simulink model "untitled1_2"  (R2020a)
settings: Solver=VariableStepAuto  StartTime=0.0  StopTime=10.0  RelTol=1e-3
values from neighbouring files (symbols this model uses):
  th1 = 3.1    [Lab1.m]
  th2 = 9.5    [Lab1.m]
  th3 = 0.24    [Lab1.m]
  th4 = 0.77    [Lab1.m]
settings Model: Creator=ajankowi  LastModifiedBy=adamj

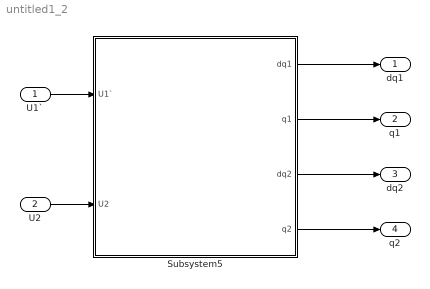
== system untitled1_2 ==
  U1` : Inport
  U2 : Inport  Port=2
  Subsystem5 : Subsystem
  dq1 : Outport
  q1 : Outport  Port=2
  dq2 : Outport  Port=3
  q2 : Outport  Port=4
  wires:
  U1`/1 -> Subsystem5/1(U1`)
  U2/1 -> Subsystem5/2(U2)
  Subsystem5/1(dq1) -> dq1/1
  Subsystem5/2(q1) -> q1/1
  Subsystem5/3(dq2) -> dq2/1
  Subsystem5/4(q2) -> q2/1

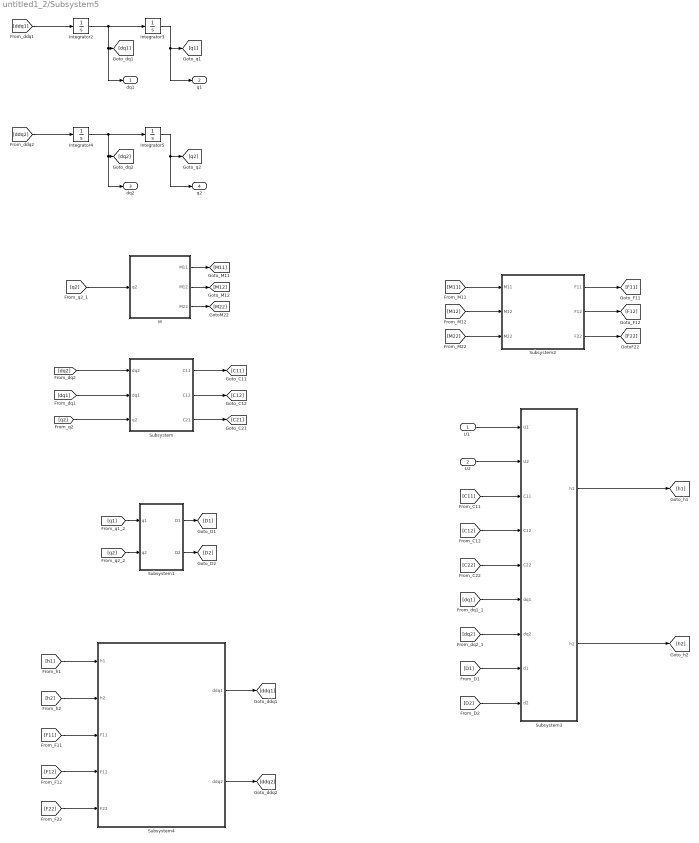
== system untitled1_2/Subsystem5 ==
  U1` : Inport
  U2 : Inport  Port=2
  Integrator{2..5} (4 alike) : Integrator
  M : Subsystem
  Subsystem : Subsystem
  Subsystem1 : Subsystem
  Subsystem2 : Subsystem
  Subsystem3 : Subsystem
  Subsystem4 : Subsystem
  dq1 : Outport
  q1 : Outport  Port=2
  dq2 : Outport  Port=3
  q2 : Outport  Port=4
  wires:
  [dq1] -> Subsystem/2(dq1)
  [q2] -> M/1(q2)
  [ddq2] -> Integrator4/1
  [D1] -> Subsystem3/8(d1)
  Integrator4/1 -> dq2/1, [dq2], Integrator5/1
  Subsystem/3(C21) -> [C21]
  [q2] -> Subsystem1/2(q2)
  Integrator2/1 -> dq1/1, [dq1], Integrator3/1
  [M22] -> Subsystem2/3(M22)
  Subsystem3/2(h2) -> [h2]
  Subsystem4/2(ddq2) -> [ddq2]
  [D2] -> Subsystem3/9(d2)
  Subsystem4/1(ddq1) -> [ddq1]
  [F11] -> Subsystem4/3(F11)
  [q1] -> Subsystem1/1(q1)
  Subsystem2/1(F11) -> [F11]
  Subsystem2/2(F12) -> [F12]
  [dq2] -> Subsystem3/7(dq2)
  [C12] -> Subsystem3/4(C12)
  [q2] -> Subsystem/3(q2)
  Subsystem1/1(D1) -> [D1]
  [h2] -> Subsystem4/2(h2)
  U1`/1 -> Subsystem3/1(U1`)
  M/1(M11) -> [M11]
  Integrator5/1 -> q2/1, [q2]
  [C22] -> Subsystem3/5(C22)
  Integrator3/1 -> q1/1, [q1]
  [dq1] -> Subsystem3/6(dq1)
  [M12] -> Subsystem2/2(M12)
  [ddq1] -> Integrator2/1
  [M11] -> Subsystem2/1(M11)
  [dq2] -> Subsystem/1(dq2)
  M/2(M12) -> [M12]
  U2/1 -> Subsystem3/2(U2)
  Subsystem/2(C12) -> [C12]
  [C11] -> Subsystem3/3(C11)
  M/3(M22) -> [M22]
  Subsystem/1(C11) -> [C11]
  Subsystem1/2(D2) -> [D2]
  Subsystem2/3(F22) -> [F22]
  [F22] -> Subsystem4/5(F22)
  [h1] -> Subsystem4/1(h1)
  [F12] -> Subsystem4/4(F12)
  Subsystem3/1(h1) -> [h1]

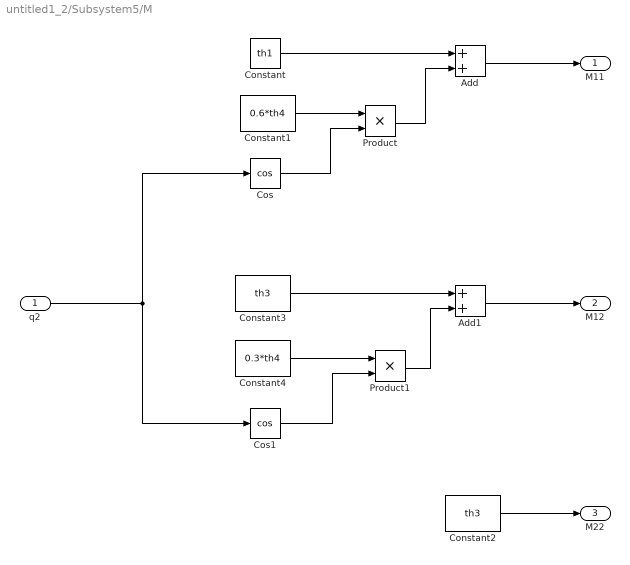
== system untitled1_2/Subsystem5/M ==
  q2 : Inport
  Add : Sum
  Add1 : Sum
  Constant : Constant  Value=th1
  Constant1 : Constant  Value=0.6*th4
  Constant2 : Constant  Value=th3
  Constant3 : Constant  Value=th3
  Constant4 : Constant  Value=0.3*th4
  Cos : Trigonometry  Operator=cos
  Cos1 : Trigonometry  Operator=cos
  Product : Product
  Product1 : Product
  M11 : Outport
  M12 : Outport  Port=2
  M22 : Outport  Port=3
  wires:
  q2/1 -> Cos/1, Cos1/1
  Constant/1 -> Add/1
  Product/1 -> Add/2
  Constant1/1 -> Product/1
  Add/1 -> M11/1
  Cos/1 -> Product/2
  Constant2/1 -> M22/1
  Add1/1 -> M12/1
  Constant3/1 -> Add1/1
  Constant4/1 -> Product1/1
  Cos1/1 -> Product1/2
  Product1/1 -> Add1/2

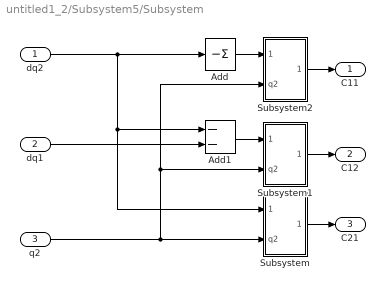
== system untitled1_2/Subsystem5/Subsystem ==
  dq2 : Inport
  dq1 : Inport  Port=2
  q2 : Inport  Port=3
  Add : Sum  Inputs=-
  Add1 : Sum  Inputs=--
  Subsystem : Subsystem
  Subsystem1 : Subsystem
  Subsystem2 : Subsystem
  C11 : Outport
  C12 : Outport  Port=2
  C21 : Outport  Port=3
  wires:
  dq2/1 -> Subsystem/1(in1), Add1/1, Add/1
  dq1/1 -> Add1/2
  q2/1 -> Subsystem2/2(q2), Subsystem1/2(q2), Subsystem/2(q2)
  Subsystem/1(out2) -> C21/1
  Add1/1 -> Subsystem1/1(in1)
  Subsystem1/1(out2) -> C12/1
  Subsystem2/1(out2) -> C11/1
  Add/1 -> Subsystem2/1(in1)

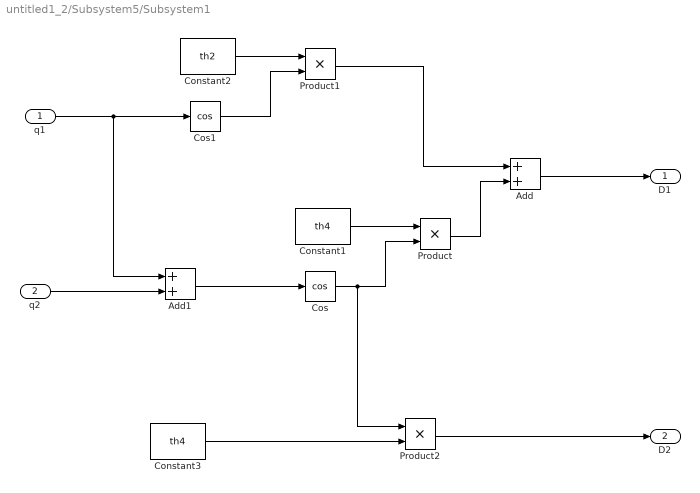
== system untitled1_2/Subsystem5/Subsystem1 ==
  q1 : Inport
  q2 : Inport  Port=2
  Add : Sum
  Add1 : Sum
  Constant1 : Constant  Value=th4
  Constant2 : Constant  Value=th2
  Constant3 : Constant  Value=th4
  Cos : Trigonometry  Operator=cos
  Cos1 : Trigonometry  Operator=cos
  Product : Product
  Product1 : Product
  Product2 : Product
  D1 : Outport
  D2 : Outport  Port=2
  wires:
  q2/1 -> Add1/2
  Constant2/1 -> Product1/1
  Constant1/1 -> Product/1
  Cos/1 -> Product2/1, Product/2
  q1/1 -> Add1/1, Cos1/1
  Product1/1 -> Add/1
  Product2/1 -> D2/1
  Add/1 -> D1/1
  Product/1 -> Add/2
  Cos1/1 -> Product1/2
  Constant3/1 -> Product2/2
  Add1/1 -> Cos/1

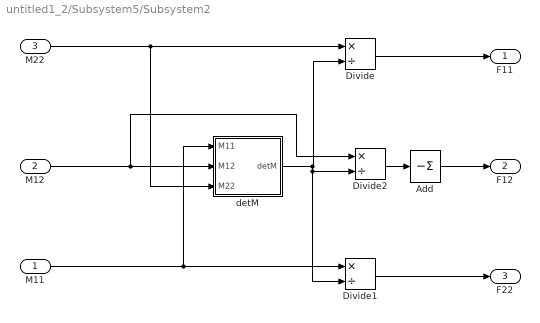
== system untitled1_2/Subsystem5/Subsystem2 ==
  M11 : Inport
  M12 : Inport  Port=2
  M22 : Inport  Port=3
  Add : Sum  Inputs=-
  Divide : Product  Inputs=*/
  Divide1 : Product  Inputs=*/
  Divide2 : Product  Inputs=*/
  detM : MATLAB Function  TreatAsAtomicUnit=on
  F11 : Outport
  F12 : Outport  Port=2
  F22 : Outport  Port=3
  wires:
  M11/1 -> Divide1/1, detM/1(M11)
  Divide1/1 -> F22/1
  Add/1 -> F12/1
  detM/1(detM) -> Divide1/2, Divide2/2, Divide/2
  M22/1 -> Divide/1, detM/3(M22)
  M12/1 -> Divide2/1, detM/2(M12)
  Divide/1 -> F11/1
  Divide2/1 -> Add/1

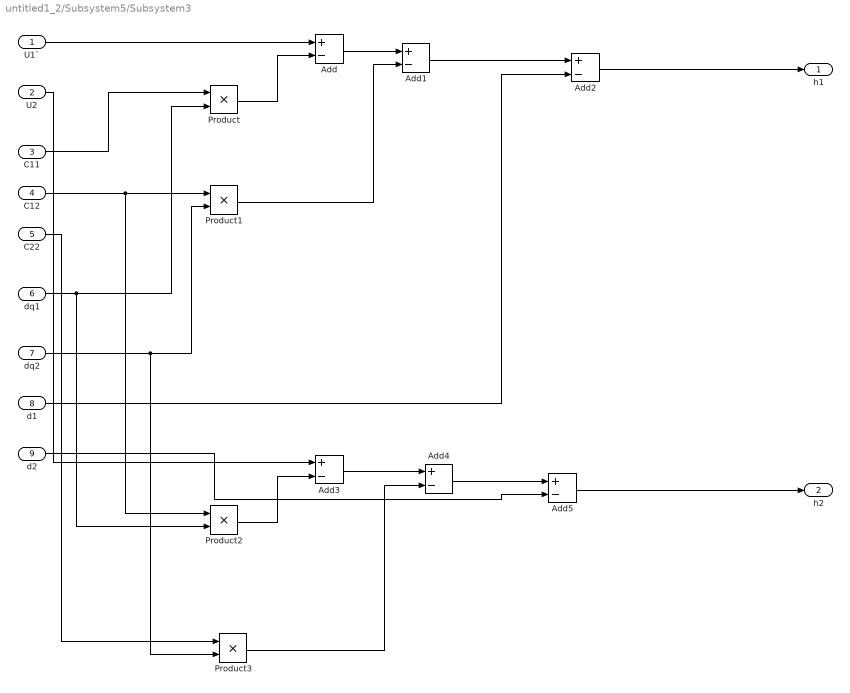
== system untitled1_2/Subsystem5/Subsystem3 ==
  U1` : Inport
  U2 : Inport  Port=2
  C11 : Inport  Port=3
  C12 : Inport  Port=4
  C22 : Inport  Port=5
  dq1 : Inport  Port=6
  dq2 : Inport  Port=7
  d1 : Inport  Port=8
  d2 : Inport  Port=9
  Add{,1..5} (6 alike) : Sum  Inputs=+-
  Product{,1..3} (4 alike) : Product
  h1 : Outport
  h2 : Outport  Port=2
  wires:
  Product/1 -> Add/2
  Add5/1 -> h2/1
  dq1/1 -> Product2/2, Product/2
  Add2/1 -> h1/1
  Add/1 -> Add1/1
  U1`/1 -> Add/1
  C22/1 -> Product3/1
  dq2/1 -> Product3/2, Product1/2
  C12/1 -> Product2/1, Product1/1
  d1/1 -> Add2/2
  Product3/1 -> Add4/2
  Product2/1 -> Add3/2
  Add1/1 -> Add2/1
  Product1/1 -> Add1/2
  d2/1 -> Add5/2
  C11/1 -> Product/1
  Add4/1 -> Add5/1
  U2/1 -> Add3/1
  Add3/1 -> Add4/1

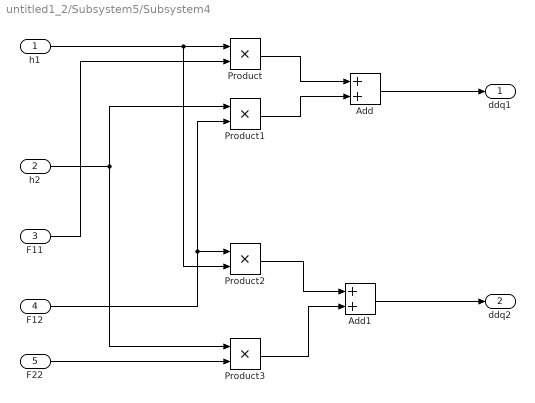
== system untitled1_2/Subsystem5/Subsystem4 ==
  h1 : Inport
  h2 : Inport  Port=2
  F11 : Inport  Port=3
  F12 : Inport  Port=4
  F22 : Inport  Port=5
  Add : Sum
  Add1 : Sum
  Product{,1..3} (4 alike) : Product
  ddq1 : Outport
  ddq2 : Outport  Port=2
  wires:
  h2/1 -> Product1/1, Product3/1
  Product1/1 -> Add/2
  F12/1 -> Product2/1, Product1/2
  Add1/1 -> ddq2/1
  Add/1 -> ddq1/1
  h1/1 -> Product2/2, Product/1
  F11/1 -> Product/2
  Product2/1 -> Add1/1
  F22/1 -> Product3/2
  Product3/1 -> Add1/2
  Product/1 -> Add/1

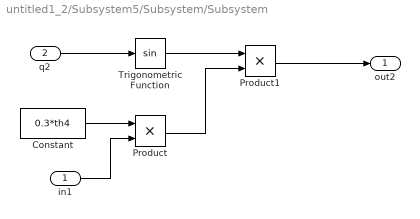
== system untitled1_2/Subsystem5/Subsystem/Subsystem ==
  in1 : Inport
  q2 : Inport  Port=2
  Constant : Constant  Value=0.3*th4
  Product : Product
  Product1 : Product
  Trigonometric Function : Trigonometry
  out2 : Outport
  wires:
  Product1/1 -> out2/1
  in1/1 -> Product/2
  Trigonometric Function/1 -> Product1/1
  q2/1 -> Trigonometric Function/1
  Product/1 -> Product1/2
  Constant/1 -> Product/1

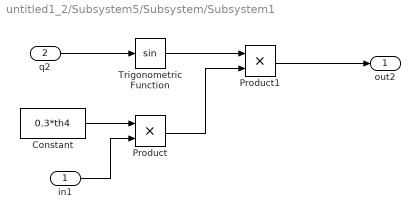
== system untitled1_2/Subsystem5/Subsystem/Subsystem1 ==
  in1 : Inport
  q2 : Inport  Port=2
  Constant : Constant  Value=0.3*th4
  Product : Product
  Product1 : Product
  Trigonometric Function : Trigonometry
  out2 : Outport
  wires:
  Product1/1 -> out2/1
  in1/1 -> Product/2
  Trigonometric Function/1 -> Product1/1
  q2/1 -> Trigonometric Function/1
  Product/1 -> Product1/2
  Constant/1 -> Product/1

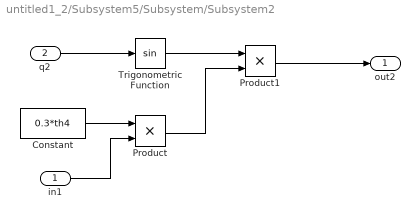
== system untitled1_2/Subsystem5/Subsystem/Subsystem2 ==
  in1 : Inport
  q2 : Inport  Port=2
  Constant : Constant  Value=0.3*th4
  Product : Product
  Product1 : Product
  Trigonometric Function : Trigonometry
  out2 : Outport
  wires:
  Product1/1 -> out2/1
  in1/1 -> Product/2
  Trigonometric Function/1 -> Product1/1
  q2/1 -> Trigonometric Function/1
  Product/1 -> Product1/2
  Constant/1 -> Product/1

== matlab function untitled1_2/Subsystem5/Subsystem2/detM ==
  data: M11 input; detM output; M12 input; M22 input
function detM = fcn(M11, M12, M22)

detM = (M11*M22)-(M12^2);
